simulink model "PM_fnc21_XloadDetection_TestHarness_backup"  (R2022a)
settings: Solver=VariableStepAuto  StartTime=0.0  StopTime=10.0  RelTol=1e-3
values from neighbouring files (symbols this model uses):
  rate_ms = 10    [PM_fnc1000_tc01_iter01_testsignal_builder.m]    (also in PM_fnc21_tc01_iter01_testsignal_builder.m; PM_fnc22_tc01_iter01_testsignal_builder.m)
settings Model: Creator=306427  LastModifiedBy=306427

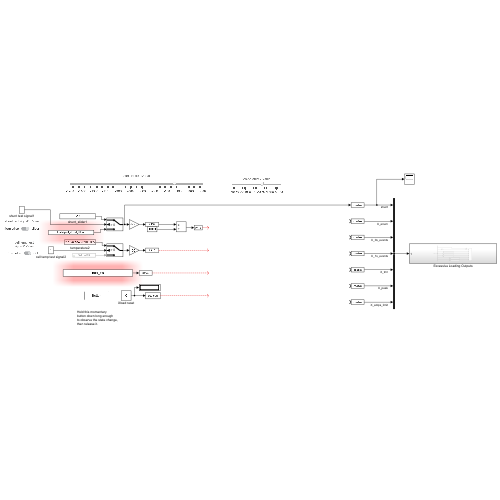
[thumbnail: Simulink's stored preview of the top-level diagram]
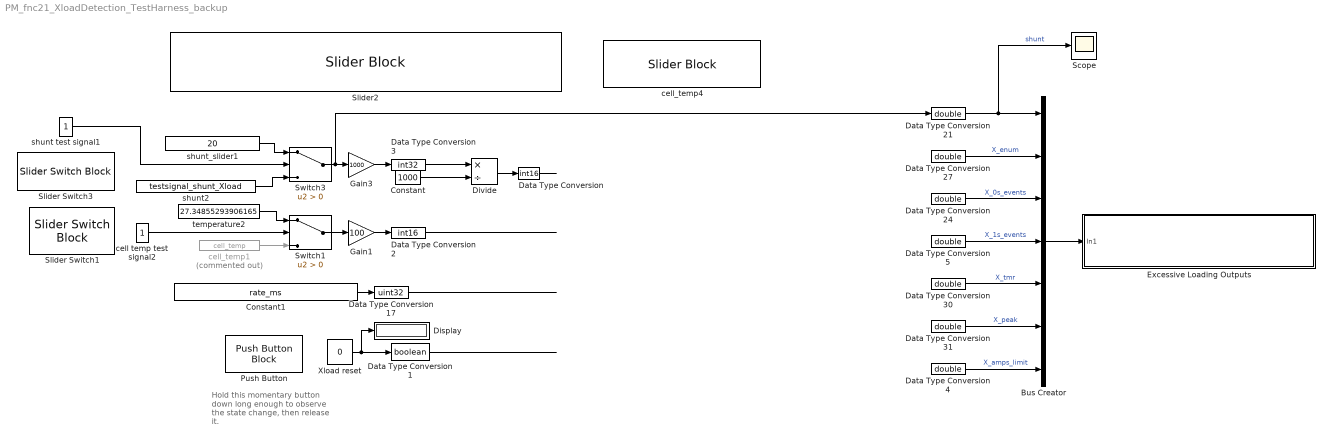
== system PM_fnc21_XloadDetection_TestHarness_backup ==
  note: Hold this momentary
      | button down long enough
      | to observe the state change,
      | then release it.
  Bus Creator : BusCreator  Inputs=7
  Constant : Constant  Value=1000
  Constant1 : Constant  Value=rate_ms
  Data Type Conversion : DataTypeConversion  OutDataTypeStr=int16  SaturateOnIntegerOverflow=off  RndMeth=Floor
  Data Type Conversion1 : DataTypeConversion  OutDataTypeStr=boolean  SaturateOnIntegerOverflow=off  RndMeth=Floor
  Data Type Conversion17 : DataTypeConversion  OutDataTypeStr=uint32  SaturateOnIntegerOverflow=off  RndMeth=Floor
  Data Type Conversion2 : DataTypeConversion  OutDataTypeStr=int16  SaturateOnIntegerOverflow=off  RndMeth=Floor
  Data Type Conversion{4..5,21,24,27,30..31} (7 alike) : DataTypeConversion  OutDataTypeStr=double  SaturateOnIntegerOverflow=off  RndMeth=Floor
  Data Type Conversion3 : DataTypeConversion  OutDataTypeStr=int32  SaturateOnIntegerOverflow=off  RndMeth=Floor
  Display : Display
  Divide : Product  Inputs=*/  OutDataTypeStr=int32  SaturateOnIntegerOverflow=on
  Excessive Loading Outputs : Subsystem
  Gain1 : Gain  Gain=100
  Gain3 : Gain  Gain=1000
  Push Button : PushButtonBlock  IconColor=On  OffValue=0.000000
  Scope : Scope
  Slider Switch1 : SliderSwitchBlock
      settings: Values={{'from wksp', 'slider'}, [0 1]}
  Slider Switch3 : SliderSwitchBlock
      settings: Values={{'from wksp', 'slider'}, [0 1]}
  Slider2 : SliderBlock  ScaleMin=-1700  ScaleMax=+500
  Switch1 : Switch  Criteria=u2 > Threshold  SaturateOnIntegerOverflow=off  InputSameDT=off
  Switch3 : Switch  Criteria=u2 > Threshold  SaturateOnIntegerOverflow=off  InputSameDT=off
  Xload reset : Constant  Value=0  OutDataTypeStr=Inherit: Inherit via back propagation
  cell temp test signal2 : Constant
  cell_temp1 : FromWorkspace  Commented=on  VariableName=cell_temp  OutDataTypeStr=double  SampleTime=[0, 1]
  cell_temp4 : SliderBlock  ScaleMin=-40  ScaleMax=70
  shunt test signal1 : Constant
  shunt2 : FromWorkspace  VariableName=testsignal_shunt_Xload  OutDataTypeStr=double
  shunt_slider1 : Constant  Value=20  OutDataTypeStr=double
  temperature2 : Constant  Value=27.34855293906165  OutDataTypeStr=double
  wires:
  Data Type Conversion24/1 -> Bus Creator/3  "X_0s_events"
  Divide/1 -> Data Type Conversion/1
  cell temp test signal2/1 -> Switch1/2
  Data Type Conversion3/1 -> Divide/1
  Constant/1 -> Divide/2
  Data Type Conversion21/1 -> Scope/1, Bus Creator/1  "shunt"
  Data Type Conversion/1 -> ?
  Data Type Conversion4/1 -> Bus Creator/7  "X_amps_limit"
  Constant1/1 -> Data Type Conversion17/1
  Data Type Conversion30/1 -> Bus Creator/5  "X_tmr"
  shunt test signal1/1 -> Switch3/2
  Data Type Conversion31/1 -> Bus Creator/6  "X_peak"
  Bus Creator/1 -> Excessive Loading Outputs/1(In1)
  cell_temp1/1 -> Switch1/3
  Switch1/1 -> Gain1/1
  temperature2/1 -> Switch1/1
  Gain3/1 -> Data Type Conversion3/1
  Data Type Conversion5/1 -> Bus Creator/4  "X_1s_events"
  Data Type Conversion1/1 -> ?
  Data Type Conversion27/1 -> Bus Creator/2  "X_enum"
  shunt2/1 -> Switch3/3
  Data Type Conversion2/1 -> ?
  Xload reset/1 -> Display/1, Data Type Conversion1/1
  Gain1/1 -> Data Type Conversion2/1
  shunt_slider1/1 -> Switch3/1
  Switch3/1 -> Data Type Conversion21/1, Gain3/1
  Data Type Conversion17/1 -> ?

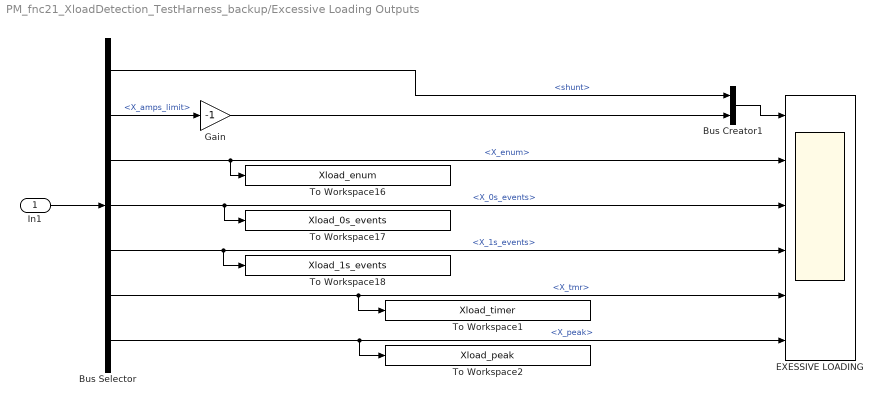
== system PM_fnc21_XloadDetection_TestHarness_backup/Excessive Loading Outputs ==
  In1 : Inport
  Bus Creator1 : BusCreator  Inputs=2
  Bus Selector : BusSelector  OutputSignals=shunt,X_amps_limit,X_enum,X_0s_events,X_1s_events,X_tmr,X_peak
  EXESSIVE LOADING : Scope  NumInputPorts=6
  Gain : Gain  Gain=-1
  To Workspace1 : ToWorkspace  VariableName=Xload_timer  SampleTime=-1
      settings: Save2DSignal=2-D array (concatenate along first dimension)
  To Workspace16 : ToWorkspace  VariableName=Xload_enum  SampleTime=-1
      settings: Save2DSignal=2-D array (concatenate along first dimension)
  To Workspace17 : ToWorkspace  VariableName=Xload_0s_events  SampleTime=-1
      settings: Save2DSignal=2-D array (concatenate along first dimension)
  To Workspace18 : ToWorkspace  VariableName=Xload_1s_events  SampleTime=-1
      settings: Save2DSignal=2-D array (concatenate along first dimension)
  To Workspace2 : ToWorkspace  VariableName=Xload_peak  SampleTime=-1
      settings: Save2DSignal=2-D array (concatenate along first dimension)
  wires:
  In1/1 -> Bus Selector/1
  Bus Selector/3 -> EXESSIVE LOADING/2, To Workspace16/1  "<X_enum>"
  Gain/1 -> Bus Creator1/2
  Bus Selector/4 -> EXESSIVE LOADING/3, To Workspace17/1  "<X_0s_events>"
  Bus Creator1/1 -> EXESSIVE LOADING/1
  Bus Selector/1 -> Bus Creator1/1  "<shunt>"
  Bus Selector/5 -> To Workspace18/1, EXESSIVE LOADING/4  "<X_1s_events>"
  Bus Selector/6 -> To Workspace1/1, EXESSIVE LOADING/5  "<X_tmr>"
  Bus Selector/7 -> To Workspace2/1, EXESSIVE LOADING/6  "<X_peak>"
  Bus Selector/2 -> Gain/1  "<X_amps_limit>"
